simulink model "zadatak1"  (R2013b)
settings: Solver=ode45  StartTime=0.0  StopTime=10  RelTol=1e-3
settings Model: Creator=KORISNIK  LastModifiedBy=KORISNIK

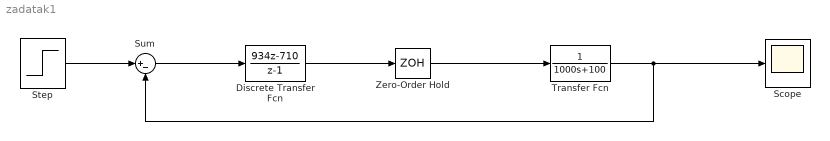
== system zadatak1 ==
  Discrete Transfer Fcn : DiscreteTransferFcn  Numerator=[934 -710]  Denominator=[1 -1]  SampleTime=0.6
  Scope : Scope
  Step : Step  SampleTime=0.01
  Sum : Sum  Inputs=|+-
  Transfer Fcn : TransferFcn  Denominator=[1000 100]
  Zero-Order Hold : ZeroOrderHold  SampleTime=0.6
  wires:
  Discrete Transfer Fcn/1 -> Zero-Order Hold/1
  Zero-Order Hold/1 -> Transfer Fcn/1
  Step/1 -> Sum/1
  Transfer Fcn/1 -> Sum/2, Scope/1
  Sum/1 -> Discrete Transfer Fcn/1
